simulink model "InvertedPendulum_DLQR_Simulink2020b"  (R2024b)
settings: Solver=ode4  StartTime=0.0  StopTime=SIM_TIME  FixedStep=STEP_SIZE  RelTol=1e-3
undefined symbols (not defined in the file): b, c, dspblkCoreblockFVToolHelper, g, gcbh, I, K_opt, l, m, M, N, theta0, theta_dot0, Ts, x0, x_dot0, x_ref0, xss
settings Model: Creator=roga  LastModifiedBy=lukas
settings SolverCC: AlgebraicLoopSolver=TrustRegion
settings DataIOCC: ReturnWorkspaceOutputs=off
settings DebuggingCC: AlgebraicLoopMsg=none  UnconnectedInputMsg=warning  UnconnectedOutputMsg=warning  UnconnectedLineMsg=warning
settings ModelReferenceCC: EnableRefExpFcnMdlSchedulingChecks=on
settings RTWCC: GPUComputeCapability=3.5  DLArmComputeVersion=19.05

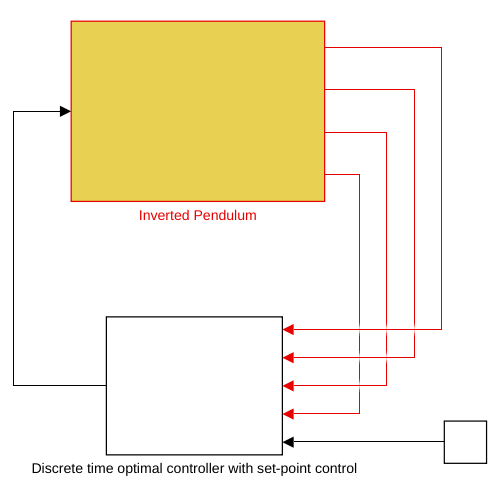
[thumbnail: Simulink's stored preview of the top-level diagram]
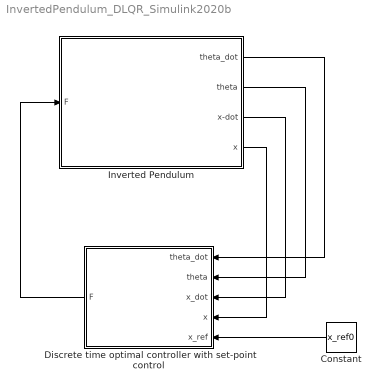
== system InvertedPendulum_DLQR_Simulink2020b ==
  Constant : Constant  Value=x_ref0  SampleTime=Ts
  Discrete time optimal controller with set-point control : Subsystem
  Inverted Pendulum : Subsystem
  wires:
  Inverted Pendulum/1(theta_dot) -> Discrete time optimal controller with set-point control/1(theta_dot)
  Inverted Pendulum/2(theta) -> Discrete time optimal controller with set-point control/2(theta)
  Inverted Pendulum/3(x-dot) -> Discrete time optimal controller with set-point control/3(x_dot)
  Inverted Pendulum/4(x) -> Discrete time optimal controller with set-point control/4(x)
  Discrete time optimal controller with set-point control/1(F) -> Inverted Pendulum/1(F)
  Constant/1 -> Discrete time optimal controller with set-point control/5(x_ref)

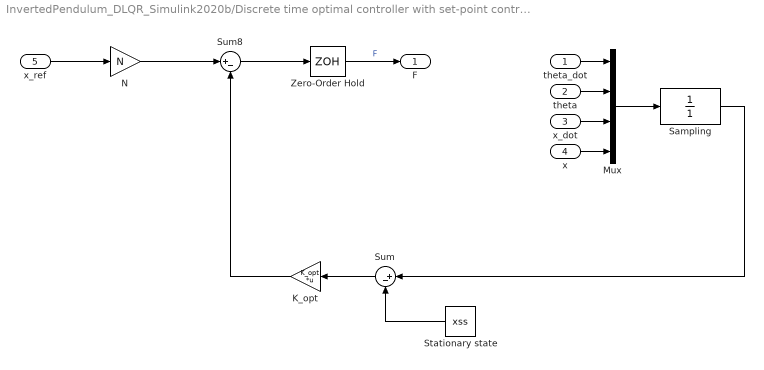
== system InvertedPendulum_DLQR_Simulink2020b/Discrete time optimal controller with set-point control ==
  theta_dot : Inport
  theta : Inport  Port=2
  x_dot : Inport  Port=3
  x : Inport  Port=4
  x_ref : Inport  Port=5
  K_opt : Gain  Gain=K_opt  Multiplication=Matrix(K*u) (u vector)
  Mux : Mux
  N : Gain  Gain=N
  Sampling : DiscreteTransferFcn  LoadFcn=dspblkCoreblockFVToolHelper(gcbh,'load');  Denominator=[1]  SampleTime=Ts
      settings: CopyFcn=dspblkCoreblockFVToolHelper(gcbh,'copy');  DeleteFcn=dspblkCoreblockFVToolHelper(gcbh,'close');  ModelCloseFcn=dspblkCoreblockFVToolHelper(gcbh,'close');  PreSaveFcn=dspblkCoreblockFVToolHelper(gcbh,'presave');  PostSaveFcn=dspblkCoreblockFVToolHelper(gcbh,'postsave');  CloseFcn=dspblkCoreblockFVToolHelper(gcbh,'close');
  Stationary state : Constant  Value=xss
  Sum : Sum  Inputs=|+-
  Sum8 : Sum  Inputs=|+-
  Zero-Order Hold : ZeroOrderHold  SampleTime=Ts
  F : Outport
  wires:
  Mux/1 -> Sampling/1
  K_opt/1 -> Sum8/2
  N/1 -> Sum8/1
  Sum/1 -> K_opt/1
  theta/1 -> Mux/2
  x/1 -> Mux/4
  Stationary state/1 -> Sum/2
  Sampling/1 -> Sum/1
  theta_dot/1 -> Mux/1
  x_dot/1 -> Mux/3
  Zero-Order Hold/1 -> F/1  "F"
  x_ref/1 -> N/1
  Sum8/1 -> Zero-Order Hold/1

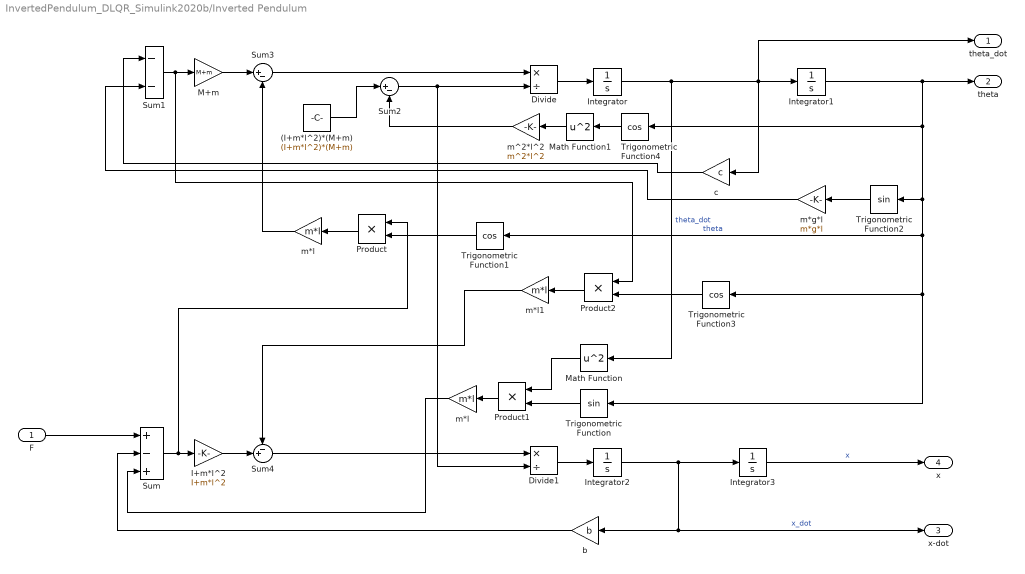
== system InvertedPendulum_DLQR_Simulink2020b/Inverted Pendulum ==
  F : Inport
  (I+m*l^2)*(M+m) : Constant  Value=(I+m*l^2)*(M+m)
  Divide : Product  Inputs=*/
  Divide1 : Product  Inputs=*/
  I+m*l^2 : Gain  Gain=I+m*l^2
  Integrator : Integrator  Priority=1  InitialCondition=theta_dot0  ContinuousStateAttributes='pendulum.angular.velocity'
  Integrator1 : Integrator  Priority=2  InitialCondition=theta0  UpperSaturationLimit=pi  LowerSaturationLimit=-pi  ContinuousStateAttributes='pendulum.angular.position'
  Integrator2 : Integrator  Priority=3  InitialCondition=x_dot0  ContinuousStateAttributes='trolley.horizontal.velocity'
  Integrator3 : Integrator  Priority=4  InitialCondition=x0  ContinuousStateAttributes='trolley.horizontal.position'
  M+m : Gain  Gain=M+m
  Math Function : Math  Operator=square
  Math Function1 : Math  Operator=square
  Product : Product
  Product1 : Product
  Product2 : Product
  Sum : Sum  Inputs=+-+
  Sum1 : Sum  Inputs=--
  Sum2 : Sum  Inputs=|+-
  Sum3 : Sum  Inputs=|+-
  Sum4 : Sum  Inputs=-+|
  Trigonometric Function : Trigonometry
  Trigonometric Function1 : Trigonometry  Operator=cos
  Trigonometric Function2 : Trigonometry
  Trigonometric Function3 : Trigonometry  Operator=cos
  Trigonometric Function4 : Trigonometry  Operator=cos
  b : Gain  Gain=b
  c : Gain  Gain=c
  m*g*l : Gain  Gain=m*g*l
  m*l : Gain  Gain=m*l
  "m*l " : Gain  Gain=m*l
  m*l1 : Gain  Gain=m*l
  m^2*l^2 : Gain  Gain=m^2*l^2
  theta_dot : Outport
  theta : Outport  Port=2
  x-dot : Outport  Port=3
  x : Outport  Port=4
  wires:
  Divide/1 -> Integrator/1
  m*l1/1 -> Sum4/1
  m*l/1 -> Sum3/2
  (I+m*l^2)*(M+m)/1 -> Sum2/1
  Math Function1/1 -> m^2*l^2/1
  Sum2/1 -> Divide1/2, Divide/2
  Divide1/1 -> Integrator2/1
  Product2/1 -> m*l1/1
  M+m/1 -> Sum3/1
  Sum4/1 -> Divide1/1
  I+m*l^2/1 -> Sum4/2
  Sum/1 -> Product/1, I+m*l^2/1
  Product1/1 -> "m*l "/1
  "m*l "/1 -> Sum/3
  Trigonometric Function2/1 -> m*g*l/1
  Integrator3/1 -> x/1  "x"
  Trigonometric Function1/1 -> Product/2
  Sum1/1 -> Product2/1, M+m/1
  Trigonometric Function3/1 -> Product2/2
  Integrator1/1 -> theta/1, Trigonometric Function4/1, Trigonometric Function2/1, Trigonometric Function1/1, Trigonometric Function3/1, Trigonometric Function/1  "theta"
  m^2*l^2/1 -> Sum2/2
  Math Function/1 -> Product1/1
  m*g*l/1 -> Sum1/2
  Trigonometric Function/1 -> Product1/2
  b/1 -> Sum/2
  Integrator2/1 -> b/1, x-dot/1, Integrator3/1  "x_dot"
  Integrator/1 -> Math Function/1, theta_dot/1, c/1, Integrator1/1  "theta_dot"
  c/1 -> Sum1/1
  Sum3/1 -> Divide/1
  Product/1 -> m*l/1
  Trigonometric Function4/1 -> Math Function1/1
  F/1 -> Sum/1
